simulink model "SimpleMass"  (R2018a)
settings: Solver=VariableStepAuto  StartTime=0.0  StopTime=Ttot  MaxStep=0.1  RelTol=1e-3
values from neighbouring files (symbols this model uses):
  DeadTimeValve = 0.05    [SimpleRotatinMass_script.m]
  droop = 0.10    (= 0.1)    [SimpleRotatinMass_script.m]
  J = 2 * H * Sn / omegan^2    (= 9524.19126238)    [SimpleRotatinMass_script.m]
  Jtwo = 2 * H * Sn / omegan^2    (= 19048.3825248)    [SimpleRotatinMass_script.m]
  omegan = 2 * pi * Fn / np    (= 314.159265359)    [SimpleRotatinMass_script.m]
  Peini = 0.26    [SimpleRotatinMass_script.m]
  Pestep = 0.12    [SimpleRotatinMass_script.m]
  RateSec = 1/20    (= 0.05)    [SimpleRotatinMass_script.m]
  Sn = 2*47e6    (= 94000000)    [SimpleRotatinMass_script.m]
  StepTime = 10    [SimpleRotatinMass_script.m]
  Tgt1 = 0.1    [SimpleRotatinMass_script.m]
  Tgt2 = 1.5    [SimpleRotatinMass_script.m]
  Tsec = 4    [SimpleRotatinMass_script.m]
  Tsec_on_delay = 40    [SimpleRotatinMass_script.m]
settings Model: Creator=daniemot  LastModifiedBy=daniemot

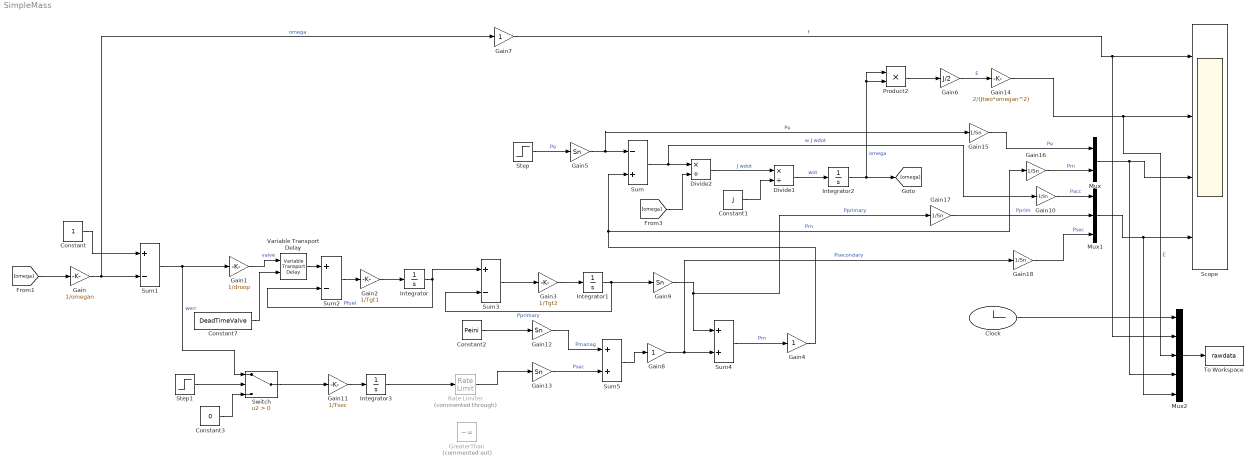
== system SimpleMass ==
  Clock : Clock
  Constant : Constant
  Constant1 : Constant  Value=J
  Constant2 : Constant  Value=Peini
  Constant3 : Constant  Value=0
  Constant7 : Constant  Value=DeadTimeValve
  Divide1 : Product  Inputs=*/
  Divide2 : Product  Inputs=*/
  Gain : Gain  Gain=1/omegan
  Gain1 : Gain  Gain=1/droop
  Gain10 : Gain  Gain=-1/Sn
  Gain11 : Gain  Gain=1/Tsec
  Gain{5,9,12..13} (4 alike) : Gain  Gain=Sn
  Gain14 : Gain  Gain=2/(Jtwo*omegan^2)
  Gain{15..18} (4 alike) : Gain  Gain=1/Sn
  Gain2 : Gain  Gain=1/Tgt1
  Gain3 : Gain  Gain=1/Tgt2
  Gain4 : Gain
  Gain6 : Gain  Gain=J/2
  Gain7 : Gain
  Gain8 : Gain
  GreaterThan : RelationalOperator  Commented=on  Operator=~=  OutDataTypeStr=boolean  RndMeth=Simplest
  Integrator : Integrator
  Integrator1 : Integrator
  Integrator2 : Integrator  InitialCondition=omegan
  Integrator3 : Integrator
  Mux : Mux  Inputs=2
  Mux1 : Mux  Inputs=3
  Mux2 : Mux  Inputs=5
  Product2 : Product
  Rate Limiter : RateLimiter  Commented=through  RisingSlewLimit=RateSec  FallingSlewLimit=-RateSec  SampleTimeMode=inherited
  Scope : Scope  NumInputPorts=4
  Step : Step  Time=StepTime  Before=Peini  After=Peini + Pestep  SampleTime=0
  Step1 : Step  Time=Tsec_on_delay  SampleTime=0
  Sum : Sum  Inputs=-+
  Sum1 : Sum  Inputs=+-
  Sum2 : Sum  Inputs=+-
  Sum3 : Sum  Inputs=+-
  Sum4 : Sum
  Sum5 : Sum
  Switch : Switch  Criteria=u2 > Threshold
  To Workspace : ToWorkspace  VariableName=rawdata  SampleTime=-1
  Variable Transport Delay : VariableTransportDelay  VariableDelayType=Variable transport delay  MaximumDelay=10  MaximumPoints=4096
  wires:
  [omega] -> Gain/1
  Gain/1 -> Sum1/2, Gain7/1  "omega"
  Constant/1 -> Sum1/1
  Sum1/1 -> Switch/1, Gain1/1  "werr"
  Gain1/1 -> Variable Transport Delay/1  "valve"
  Gain2/1 -> Integrator/1
  Sum2/1 -> Gain2/1
  Integrator1/1 -> Gain9/1, Sum3/2  "Pprimary"
  Integrator/1 -> Sum3/1, Sum2/2  "Pfuel"
  Gain3/1 -> Integrator1/1
  Sum3/1 -> Gain3/1
  Gain4/1 -> Gain16/1, Sum/2  "Pm"
  Step/1 -> Gain5/1  "Pe"
  Gain5/1 -> Gain15/1, Sum/1  "Pe"
  Divide2/1 -> Divide1/1  "J wdot"
  Constant1/1 -> Divide1/2
  Divide1/1 -> Integrator2/1  "wot"
  Integrator2/1 -> Product2/2, Product2/1, [omega]  "omega"
  Product2/1 -> Gain6/1
  Constant2/1 -> Gain12/1
  Sum4/1 -> Gain4/1  "Pm"
  [omega] -> Divide2/2
  Sum/1 -> Gain10/1, Divide2/1  "w J wdot"
  Gain6/1 -> Gain14/1  "E"
  Variable Transport Delay/1 -> Sum2/1
  Constant7/1 -> Variable Transport Delay/2
  Gain7/1 -> Mux2/2, Scope/1  "f"
  Gain8/1 -> Gain18/1, Sum4/2  "Psecondary"
  Gain9/1 -> Gain17/1, Sum4/1  "Pprimary"
  Sum5/1 -> Gain8/1
  Gain11/1 -> Integrator3/1
  Rate Limiter/1 -> Gain13/1
  Mux/1 -> Mux2/4, Scope/3
  Gain10/1 -> Mux1/1  "Pacc"
  Mux1/1 -> Mux2/5, Scope/4
  Gain12/1 -> Sum5/1  "Pmanag"
  Gain13/1 -> Sum5/2  "Psec"
  Integrator3/1 -> Rate Limiter/1
  Switch/1 -> Gain11/1
  Step1/1 -> Switch/2
  Constant3/1 -> Switch/3
  Gain14/1 -> Mux2/3, Scope/2  "E"
  Gain15/1 -> Mux/1  "Pe"
  Gain16/1 -> Mux/2  "Pm"
  Gain17/1 -> Mux1/2  "Pprim"
  Gain18/1 -> Mux1/3  "Psec"
  Mux2/1 -> To Workspace/1
  Clock/1 -> Mux2/1
